simulink model "SumFilter"  (R2019b)
settings: Solver=VariableStepAuto  StartTime=0.0  StopTime=SimTime  RelTol=1e-3
values from neighbouring files (symbols this model uses):
  Denominator = [R*C 1]    [Script.m]
  Numerator = [1]    [Script.m]
settings Model: Creator=Illia Bannitsyn  LastModifiedBy=Illia Bannitsyn

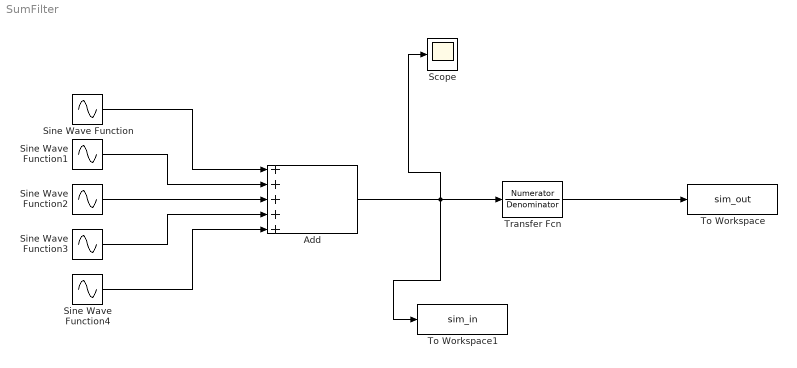
== system SumFilter ==
  Add : Sum  Inputs=+++++
  Scope : Scope
  Sine Wave Function : Sin  Amplitude=2  Frequency=0.01  Phase=1  SampleTime=0
  Sine Wave Function1 : Sin  Amplitude=3  Phase=5  SampleTime=0
  Sine Wave Function2 : Sin  Frequency=30  Phase=5  SampleTime=0
  Sine Wave Function3 : Sin  Amplitude=2  Frequency=0.01  Phase=1  SampleTime=0
  Sine Wave Function4 : Sin  Amplitude=4  Frequency=5  SampleTime=0
  To Workspace : ToWorkspace  VariableName=sim_out  SaveFormat=Timeseries  SampleTime=-1
  To Workspace1 : ToWorkspace  VariableName=sim_in  SaveFormat=Timeseries  SampleTime=-1
  Transfer Fcn : TransferFcn  Numerator=Numerator  Denominator=Denominator
  wires:
  Sine Wave Function/1 -> Add/1
  Sine Wave Function1/1 -> Add/2
  Sine Wave Function2/1 -> Add/3
  Sine Wave Function3/1 -> Add/4
  Sine Wave Function4/1 -> Add/5
  Add/1 -> Scope/1, To Workspace1/1, Transfer Fcn/1
  Transfer Fcn/1 -> To Workspace/1
